simulink model "Over_Voltage"  (R2017a)
settings: Solver=VariableStepAuto  StartTime=0.0  StopTime=10.0  MaxStep=1e-4  RelTol=1e-3
libraries: powerlib x8, powerlib_meascontrol x4, simulink_extras x3
settings Model: Creator=ikon  LastModifiedBy=ikon

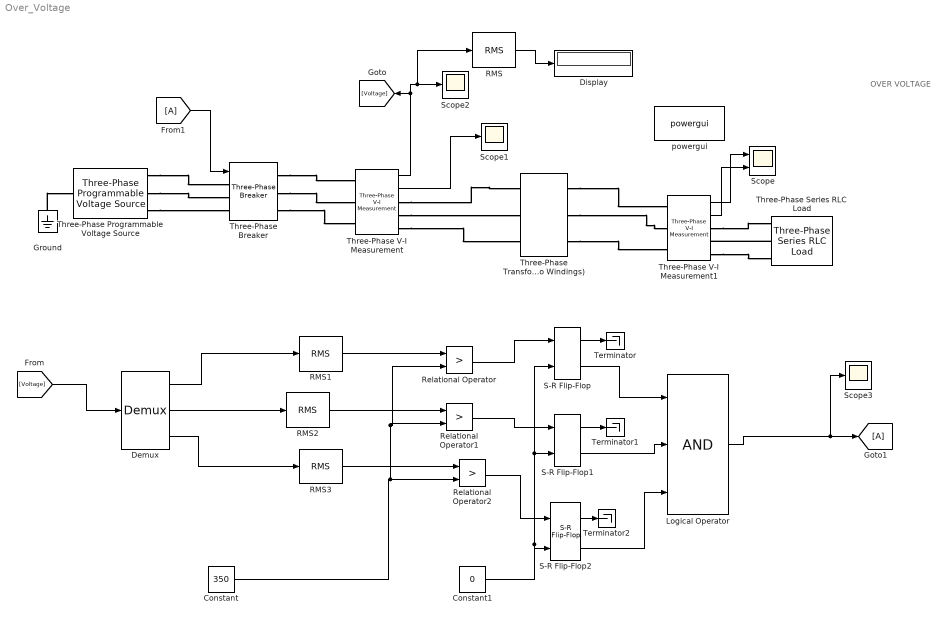
== system Over_Voltage ==
  note: OVER VOLTAGE
  Constant : Constant  Value=350
  Constant1 : Constant  Value=0  OutDataTypeStr=boolean
  Demux : Demux  Outputs=3
  Display : Display
  Ground : powerlib/Elements/Ground  LConnTagsString=a
  Logical Operator : Logic  Inputs=3  AllPortsSameDT=off  OutDataTypeStr=boolean
  RMS{,1..3} (4 alike) : powerlib_meascontrol/Measurements/RMS  TrueRMS=on  Freq=60  RMSInit=120  Ts=0
  Relational Operator : RelationalOperator  Operator=>  OutDataTypeStr=boolean  RndMeth=Simplest
  Relational Operator1 : RelationalOperator  Operator=>  OutDataTypeStr=boolean  RndMeth=Simplest
  Relational Operator2 : RelationalOperator  Operator=>  OutDataTypeStr=boolean  RndMeth=Simplest
  S-R Flip-Flop : simulink_extras/Flip Flops/S-R Flip-Flop  initial_condition=0
  S-R Flip-Flop1 : simulink_extras/Flip Flops/S-R Flip-Flop  initial_condition=0
  S-R Flip-Flop2 : simulink_extras/Flip Flops/S-R Flip-Flop  initial_condition=0
  Scope : Scope  NumInputPorts=2
  Scope1 : Scope
  Scope2 : Scope
  Scope3 : Scope
  Terminator : Terminator
  Terminator1 : Terminator
  Terminator2 : Terminator
  Three-Phase Programmable Voltage Source : powerlib/Electrical Sources/Three-Phase Programmable Voltage Source  PositiveSequence="[400  0 50]"  VariationEntity=Amplitude  VariationType=Table of time-amplitude pairs  VariationTypeAlt=Step  VariationStep=0.5  VariationRate=10  VariationMagnitude=0.3  VariationFrequency=2  VariationTiming=[1 2]  VariationPhaseA=off  Amplitudes=[1 1.2 1.5]  TimeValues="[0 2  3]"  HarmonicGeneration=off  HarmonicA=[3 0.2 -25 0]  HarmonicB=[2 0.15 35 2]  Timing="[0.05  3]"  BusType=swing  Pref=0  Qref=0  Qmin=-inf  Qmax=inf
  Three-Phase Series RLC Load : powerlib/Elements/Three-Phase Series RLC Load  LConnTagsString=A|B|C  Configuration=Y (grounded)  NominalVoltage=1000  Vabc=[1e3 1e3 1e3]  Vabcp=[1e3 1e3 1e3]  NominalFrequency=50  UnbalancedPower=off  ActivePower=10e3  InductivePower=100  CapacitivePower=100  Pabc=[10e3 9e3 11e3]  QLabc=[100 90 110]  QCabc=[100 90 110]  Pabcp=[10e3 9e3 11e3]  QLabcp=[100 90 110]  QCabcp=[100 90 110]  Measurements=None  LoadType=constant Z
  Three-Phase Transformer (Two Windings) : powerlib/Elements/Three-Phase Transformer (Two Windings)  Winding1Connection=Yg  Winding2Connection=Yg  CoreType=Three single-phase transformers  SetSaturation=off  Hysteresis=off  DataFile='hysteresis'  SetInitialFlux=off  Measurements=None  UNITS=pu  NominalPower=[ 250e6 , 60 ]  Winding1=[ 735e3 , 0.002 , 0.08 ]  Winding2=[ 315e3 , 0.002 , 0.08 ]  Rm=500  Lm=500  L0=0.5  Saturation=[ 0,0 ; 0.0024,1.2 ; 1.0,1.52 ]  InitialFluxes=[ 0.8 , -0.8 , 0.7 ]  MoreParameters=off  BreakLoop=off  DataType=off  TransfoNumber=1
  Three-Phase V-I Measurement : powerlib/Measurements/Three-Phase V-I Measurement  VoltageMeasurement=phase-to-ground  SetLabelV=off  LabelV=Vabc  Vpu=off  VpuLL=off  CurrentMeasurement=yes  SetLabelI=off  LabelI=Iabc  Ipu=off  Pbase=100e6  Vbase=500e3  OutputType=Complex  PhasorSimulation=off  PSBequivalent=0
  Three-Phase V-I Measurement1 : powerlib/Measurements/Three-Phase V-I Measurement  VoltageMeasurement=phase-to-ground  SetLabelV=off  LabelV=Vabc  Vpu=off  VpuLL=off  CurrentMeasurement=yes  SetLabelI=off  LabelI=Iabc  Ipu=off  Pbase=100e6  Vbase=500e3  OutputType=Complex  PhasorSimulation=off  PSBequivalent=0
  Three-Phase Breaker : powerlib/Elements/Three-Phase Breaker  InitialState=closed  SwitchA=on  SwitchB=on  SwitchC=on  SwitchTimes="[1/60  5/60]"  External=on  BreakerResistance=0.001  SnubberResistance=1e6  SnubberCapacitance=inf  Measurements=None
  powergui : powerlib/powergui  Priority=1  SimulationMode=Continuous  SampleTime=50e-6  frequency=60  Iterations=50  frequencyindice=50  Pbase=100e6  ErrMax=1e-4  UnitsV=kV  UnitsW=MW  buscounter=0  FunctionMessages=off  echomessages=off  EnableUseOfTLC=off  CurrentSourceSwitches=off  DisableSnubberDevices=off  DisableRonSwitches=off  DisableVfSwitches=off  DisplayEquations=off  SolverType=Tustin/Backward Euler (TBE)  Interpol=off  ExternalGateDelay=off  methode=off  Ts=100  x0status=blocks  SPID=on  SwTol=0  HookPort=off  RestoreLinks=warning  ResistiveCurrentMeasurement=off  Frange=[0:2:500]  Ylog=off  Xlog=on  ShowGrid=off  save=off  variable=ZData  structure=0  ZoomFFT=off  StartTime=0.0  cycles=1  DisplayStyle=1  fundamental=60  FreqAxis=off  MaxFrequency=1000  frequencyindicesteady=1  RmsSteady=1  display=off
  wires:
  Three-Phase V-I Measurement1/1 -> Scope/1
  Three-Phase V-I Measurement1/2 -> Scope/2
  Three-Phase V-I Measurement/2 -> Scope1/1
  Three-Phase V-I Measurement/1 -> [Voltage], RMS/1, Scope2/1
  RMS/1 -> Display/1
  [Voltage] -> Demux/1
  Demux/1 -> RMS1/1
  Demux/2 -> RMS2/1
  Demux/3 -> RMS3/1
  RMS2/1 -> Relational Operator1/1
  RMS1/1 -> Relational Operator/1
  RMS3/1 -> Relational Operator2/1
  Constant/1 -> Relational Operator/2, Relational Operator1/2, Relational Operator2/2
  Relational Operator2/1 -> S-R Flip-Flop2/1
  Relational Operator1/1 -> S-R Flip-Flop1/1
  Relational Operator/1 -> S-R Flip-Flop/1
  Constant1/1 -> S-R Flip-Flop2/2, S-R Flip-Flop1/2, S-R Flip-Flop/2
  S-R Flip-Flop/2 -> Logical Operator/1
  S-R Flip-Flop1/2 -> Logical Operator/2
  S-R Flip-Flop2/2 -> Logical Operator/3
  S-R Flip-Flop/1 -> Terminator/1
  S-R Flip-Flop1/1 -> Terminator1/1
  S-R Flip-Flop2/1 -> Terminator2/1
  Logical Operator/1 -> [A], Scope3/1
  [A] -> Three-Phase Breaker/1
  connections:
  Ground/LConn1 -- Three-Phase Programmable Voltage Source/LConn1
  Three-Phase Series RLC Load/LConn2 -- Three-Phase V-I Measurement1/RConn2
  Three-Phase V-I Measurement1/RConn1 -- Three-Phase Series RLC Load/LConn1
  Three-Phase V-I Measurement1/RConn3 -- Three-Phase Series RLC Load/LConn3
  Three-Phase Transformer (Two Windings)/RConn1 -- Three-Phase V-I Measurement1/LConn1
  Three-Phase Transformer (Two Windings)/RConn2 -- Three-Phase V-I Measurement1/LConn2
  Three-Phase Transformer (Two Windings)/RConn3 -- Three-Phase V-I Measurement1/LConn3
  Three-Phase V-I Measurement/RConn1 -- Three-Phase Transformer (Two Windings)/LConn1
  Three-Phase V-I Measurement/RConn2 -- Three-Phase Transformer (Two Windings)/LConn2
  Three-Phase V-I Measurement/RConn3 -- Three-Phase Transformer (Two Windings)/LConn3
  Three-Phase Programmable Voltage Source/RConn2 -- Three-Phase Breaker/LConn2
  Three-Phase Programmable Voltage Source/RConn3 -- Three-Phase Breaker/LConn3
  Three-Phase Programmable Voltage Source/RConn1 -- Three-Phase Breaker/LConn1
  Three-Phase Breaker/RConn1 -- Three-Phase V-I Measurement/LConn1
  Three-Phase Breaker/RConn2 -- Three-Phase V-I Measurement/LConn2
  Three-Phase Breaker/RConn3 -- Three-Phase V-I Measurement/LConn3
